simulink model "Arduino_Encoder"  (R2015b)
settings: Solver=VariableStepAuto  StartTime=0.0  StopTime=10  RelTol=1e-3
libraries: arduino_io_lib x3
settings Model: Creator=es2lab2  LastModifiedBy=es2lab2
settings GRTTargetCC: ExtMode=on  ExtModeTransport=1  ExtModeMexFile=ext_serial_win32_comm

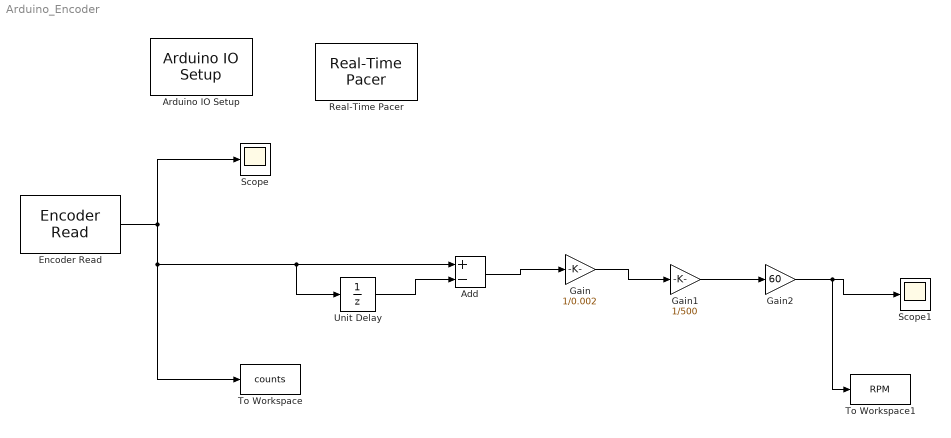
== system Arduino_Encoder ==
  Add : Sum  Inputs=+-
  Arduino IO Setup : arduino_io_lib/Arduino IO Setup  Priority=3  arduinoVar=Temporary arduino variable: Arduino1  workspaceVarName=a  comPort=COM118
  Encoder Read : arduino_io_lib/Encoder Read  arduinoVar=Temporary arduino variable: Arduino1  encNum=1  pinA=2  pinB=3  DbDl=0  T=0.002
  Gain : Gain  Gain=1/0.002
  Gain1 : Gain  Gain=1/500
  Gain2 : Gain  Gain=60
  Real-Time Pacer : arduino_io_lib/Real-Time Pacer  simTimePerRealTime=1
  Scope : Scope
  Scope1 : Scope
  To Workspace : ToWorkspace  VariableName=counts  SaveFormat=Timeseries  SampleTime=-1
  To Workspace1 : ToWorkspace  VariableName=RPM  SaveFormat=Timeseries  SampleTime=-1
  Unit Delay : UnitDelay  SampleTime=-1
  wires:
  Encoder Read/1 -> Unit Delay/1, Add/1, To Workspace/1, Scope/1
  Unit Delay/1 -> Add/2
  Add/1 -> Gain/1
  Gain/1 -> Gain1/1
  Gain1/1 -> Gain2/1
  Gain2/1 -> To Workspace1/1, Scope1/1
